simulink model "ErlangSEIRv2_4"  (R2019b)
settings: Solver=VariableStepAuto  StartTime=0.0  StopTime=365  FixedStep=1/24  RelTol=1e-12
undefined symbols (not defined in the file or in its folder): sigbuilder_block
libraries: simulink x2
settings Model: OrderedModelArguments=off  Creator=Alex  LastModifiedBy=Alex

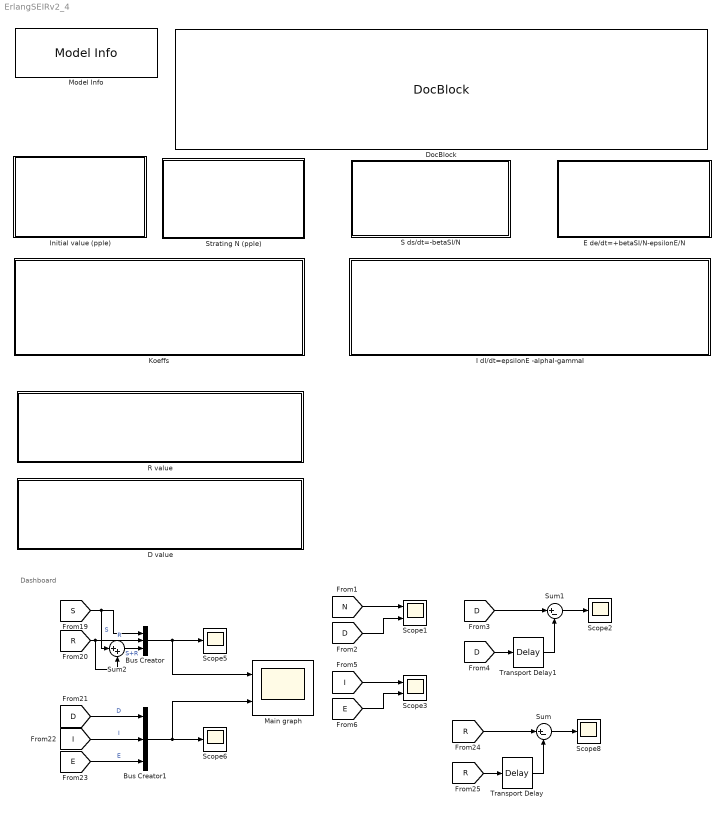
== system ErlangSEIRv2_4 ==
  note: Dashboard
  Bus Creator : BusCreator  Inputs=3
  Bus Creator1 : BusCreator  Inputs=3
  D value : Subsystem
  DocBlock : simulink/Model-Wide Utilities/DocBlock  DocumentType=Text
      content=|
      | Классическая SEIR модель с учетом рождаемости и естественной смертности
      |
      | Учитываются колебания r0 за сутки (часовые ритмы), недельные, месячные (30) дней, и квартальные
      | Ритмы моделируются через синусоиды соответствующего периода (1, 7, 30, 120)
      |
      | Подключен нормально распределенный источник случайностей, частота генерации чисел - 1 день
      |
      | Малое население 1470
      |
      | Учтены ограничительные меры (переключением поправок в Signal Builder)
      | вторая волна не моделируется ввиду исчерпания населения???
      |
      | Для статьи в Резекне 2021
      |
      | На базе этой модели строятся последующие вариации
  E de/dt=+betaSI/N-epsilonE/N : Subsystem
  I dI/dt=epsilonE -alphaI-gammaI : Subsystem
  Initial value (pple) : Subsystem
  Koeffs : Subsystem
  Main graph : Scope  NumInputPorts=2
  Model Info : simulink/Model-Wide Utilities/Model Info  Frame=on  DisplayStringWithTags=|  HorizontalTextAlignment=Left  LeftAlignmentValue=0.02
      | Информация
      | %<Created>
      | %<ModelVersion>
      | %<Description>
  R value : Subsystem
  S ds/dt=-betaSI/N : Subsystem
  Scope1 : Scope  NumInputPorts=2
  Scope{2,5..6,8} (4 alike) : Scope
  Scope3 : Scope  NumInputPorts=2
  Strating N (pple) : Subsystem
  Sum : Sum  Inputs=|+-
  Sum1 : Sum  Inputs=|+-
  Sum2 : Sum  Inputs=|++
  Transport Delay : TransportDelay
  Transport Delay1 : TransportDelay
  wires:
  [S] -> Sum2/1, Bus Creator/1  "S"
  [R] -> Sum2/2, Bus Creator/2  "R"
  [D] -> Bus Creator1/1  "D"
  [I] -> Bus Creator1/2  "I"
  [E] -> Bus Creator1/3  "E"
  Bus Creator/1 -> Main graph/1, Scope5/1
  Bus Creator1/1 -> Main graph/2, Scope6/1
  [R] -> Transport Delay/1
  [R] -> Sum/1
  Transport Delay/1 -> Sum/2
  Sum/1 -> Scope8/1
  [N] -> Scope1/1
  [D] -> Scope1/2
  Sum1/1 -> Scope2/1
  Transport Delay1/1 -> Sum1/2
  [D] -> Sum1/1
  [D] -> Transport Delay1/1
  Sum2/1 -> Bus Creator/3  "S+R"
  [E] -> Scope3/2
  [I] -> Scope3/1

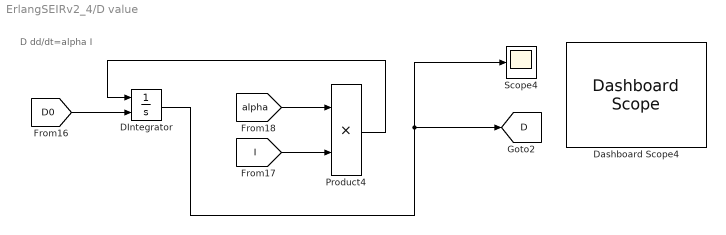
== system ErlangSEIRv2_4/D value ==
  note: D dd/dt=alpha I
  DIntegrator : Integrator  InitialConditionSource=external
  Dashboard Scope4 : DashboardScope  Ymax=150e6
  Product4 : Product  Inputs=**
  Scope4 : Scope
  tag scope: D=global
  wires:
  DIntegrator/1 -> [D], Scope4/1
  [I] -> Product4/2
  [alpha] -> Product4/1
  Product4/1 -> DIntegrator/1
  [D0] -> DIntegrator/2

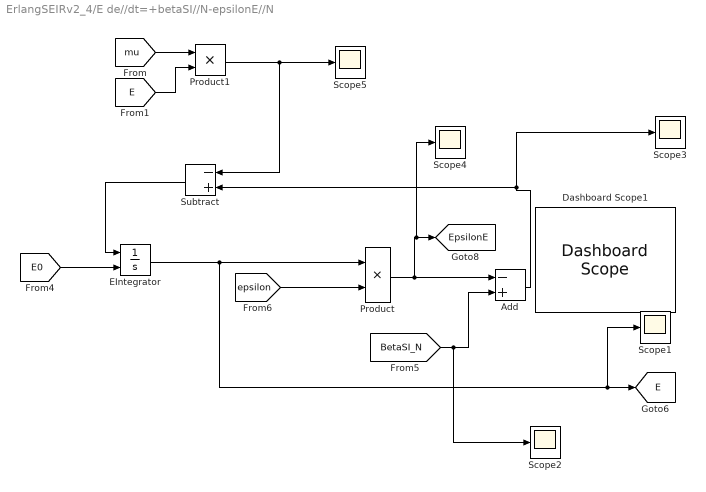
== system ErlangSEIRv2_4/E de//dt=+betaSI//N-epsilonE//N ==
  Add : Sum  Inputs=-+
  Dashboard Scope1 : DashboardScope
  EIntegrator : Integrator  InitialConditionSource=external
  Product : Product  Inputs=**
  Product1 : Product
  Scope{1..5} (5 alike) : Scope
  Subtract : Sum  Inputs=-+
  tag scope: E=global, EpsilonE=global
  wires:
  EIntegrator/1 -> Scope1/1, [E], Product/1
  [BetaSI_N] -> Scope2/1, Add/2
  Add/1 -> Subtract/2, Scope3/1
  [epsilon] -> Product/2
  Product/1 -> Scope4/1, [EpsilonE], Add/1
  [E0] -> EIntegrator/2
  [mu] -> Product1/1
  [E] -> Product1/2
  Subtract/1 -> EIntegrator/1
  Product1/1 -> Scope5/1, Subtract/1

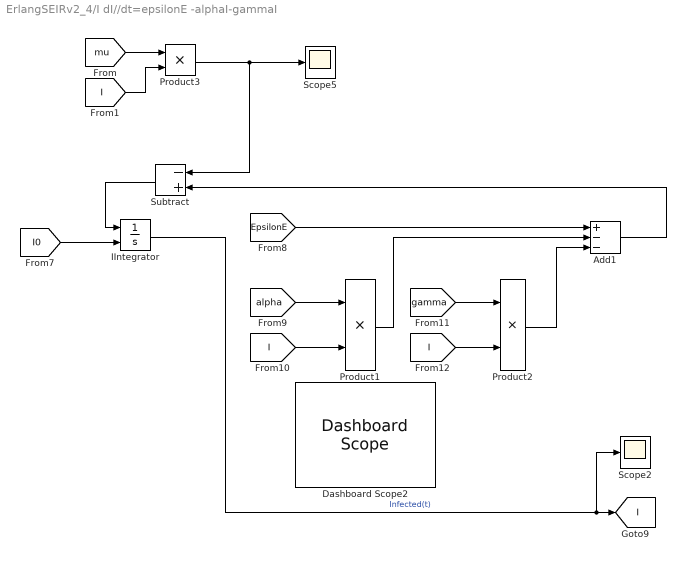
== system ErlangSEIRv2_4/I dI//dt=epsilonE -alphaI-gammaI ==
  Add1 : Sum  Inputs=+--
  Dashboard Scope2 : DashboardScope  Ymax=150e6
  IIntegrator : Integrator  InitialConditionSource=external
  Product1 : Product  Inputs=**
  Product2 : Product  Inputs=**
  Product3 : Product
  Scope2 : Scope
  Scope5 : Scope
  Subtract : Sum  Inputs=-+
  tag scope: I=global
  wires:
  [gamma] -> Product2/1
  Product2/1 -> Add1/3
  [EpsilonE] -> Add1/1
  [alpha] -> Product1/1
  Product1/1 -> Add1/2
  IIntegrator/1 -> [I], Scope2/1  "Infected(t)"
  [I] -> Product1/2
  Add1/1 -> Subtract/2
  [I] -> Product2/2
  [I0] -> IIntegrator/2
  [I] -> Product3/2
  Product3/1 -> Scope5/1, Subtract/1
  [mu] -> Product3/1
  Subtract/1 -> IIntegrator/1

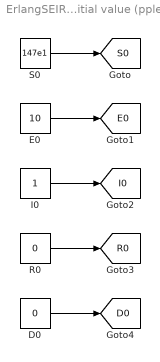
== system ErlangSEIRv2_4/Initial value (pple) ==
  D0 : Constant  Value=0
  E0 : Constant  Value=10
  I0 : Constant
  R0 : Constant  Value=0
  S0 : Constant  Value=147e1
  tag scope: D0=global, E0=global, I0=global, R0=global, S0=global
  wires:
  S0/1 -> [S0]
  I0/1 -> [I0]
  D0/1 -> [D0]
  E0/1 -> [E0]
  R0/1 -> [R0]

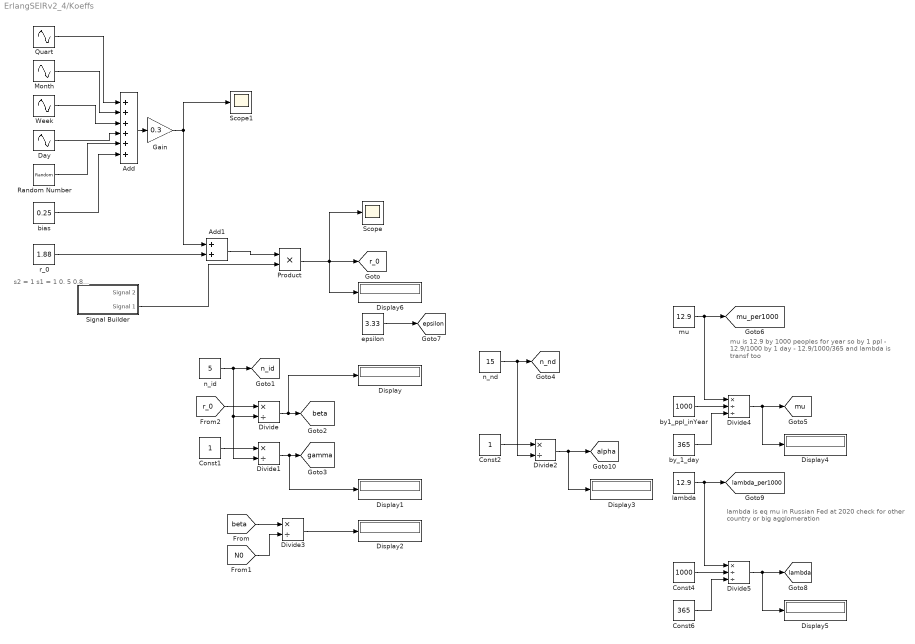
== system ErlangSEIRv2_4/Koeffs ==
  note: s2 = 1
      | s1 = 1 0. 5 0.8...
  note: lambda is eq mu in Russian Fed at 2020
      | check for other country or big agglomeration
  note: mu is 12.9 by 1000 peoples for year
      | so by 1 ppl - 12.9/1000
      | by 1 day - 12.9/1000/365
      | and lambda is transf too
  Add : Sum  Inputs=++++++
  Add1 : Sum
  Const1 : Constant
  Const2 : Constant
  Const4 : Constant  Value=1000
  Const6 : Constant  Value=365
  Day : Sin  Amplitude=0.12  Frequency=2*pi/7  SampleTime=0
  Display{,1..6} (7 alike) : Display
  Divide{,1..3} (4 alike) : Product  Inputs=*/
  Divide4 : Product  Inputs=*//
  Divide5 : Product  Inputs=*//
  Gain : Gain  Gain=0.3
  Month : Sin  Amplitude=0.12  Frequency=2*pi/30  SampleTime=0
  Product : Product
  Quart : Sin  Amplitude=0.12  Frequency=2*pi/120  SampleTime=0
  Random Number : RandomNumber  Variance=0.0144  SampleTime=1
  Scope : Scope
  Scope1 : Scope
  Signal Builder : Subsystem  Tag=STV Subsys  LoadFcn=sigbuilder_block('load');  StartFcn=sigbuilder_block('start');  StopFcn=sigbuilder_block('stop');  ClipboardFcn=sigbuilder_block('clipboard');  mask(Sigbuilder block){tuvar=[0:10]}
      mask help: Simulink:masks:SigbuilderBlock_MD
      mask init:
      | if ~strcmp(get_param(bdroot(gcbh),'SimulationStatus'),'stopped') tuvar = sigbuilder_block('maskInit'); end
      settings: CopyFcn=sigbuilder_block('copy');  DeleteFcn=sigbuilder_block('delete');  ModelCloseFcn=sigbuilder_block('modelClose');  PreSaveFcn=sigbuilder_block('preSave');  PauseFcn=sigbuilder_block('pause');  ContinueFcn=sigbuilder_block('continue');  NameChangeFcn=sigbuilder_block('namechange');  OpenFcn=sigbuilder_block('open',[437.6 199.2 550.4 400 ]);  CloseFcn=sigbuilder_block('close');
      mask Display: plot(0, 0, 100, 100,[2, 2, 32, 32, 2], [68, 8, 8, 68, 68],[32, 2], [38, 38], [32, 19, 2],[53, 60, 44], [32, 17, 17, 2],[16, 16, 31, 31]);txt = getActiveGroup(gcbh);text(2, 100, txt,'verticalAlignment', 'top');
  Week : Sin  Amplitude=0.12  Frequency=2*pi/7  SampleTime=0
  bias : Constant  Value=0.25
  by1_ppl_inYear : Constant  Value=1000
  by_1_day : Constant  Value=365
  epsilon : Constant  Value=3.33
  lambda : Constant  Value=12.9
  mu : Constant  Value=12.9
  n_id : Constant  Value=5
  n_nd : Constant  Value=15
  r_0 : Constant  Value=1.88
  tag scope: alpha=global, beta=global, epsilon=global, gamma=global, lambda=global, lambda_per1000=global, mu=global, mu_per1000=global, n_id=global, n_nd=global, r_0=global
  wires:
  Divide1/1 -> Display1/1, [gamma]
  n_id/1 -> Divide1/2, Divide/2, [n_id]
  Divide/1 -> Display/1, [beta]
  Const1/1 -> Divide1/1
  epsilon/1 -> [epsilon]
  Const2/1 -> Divide2/1
  Divide2/1 -> Display3/1, [alpha]
  n_nd/1 -> [n_nd], Divide2/2
  [beta] -> Divide3/1
  [N0] -> Divide3/2
  Divide3/1 -> Display2/1
  mu/1 -> Divide4/1, [mu_per1000]
  Divide4/1 -> [mu], Display4/1
  by1_ppl_inYear/1 -> Divide4/2
  Const4/1 -> Divide5/2
  Divide5/1 -> Display5/1, [lambda]
  lambda/1 -> [lambda_per1000], Divide5/1
  Const6/1 -> Divide5/3
  by_1_day/1 -> Divide4/3
  r_0/1 -> Add1/2
  Product/1 -> Scope/1, Display6/1, [r_0]
  [r_0] -> Divide/1
  Quart/1 -> Add/1
  Month/1 -> Add/2
  Week/1 -> Add/3
  Day/1 -> Add/4
  Add/1 -> Gain/1
  Add1/1 -> Product/1
  Random Number/1 -> Add/5
  bias/1 -> Add/6
  Gain/1 -> Scope1/1, Add1/1
  Signal Builder/2(Signal 1) -> Product/2

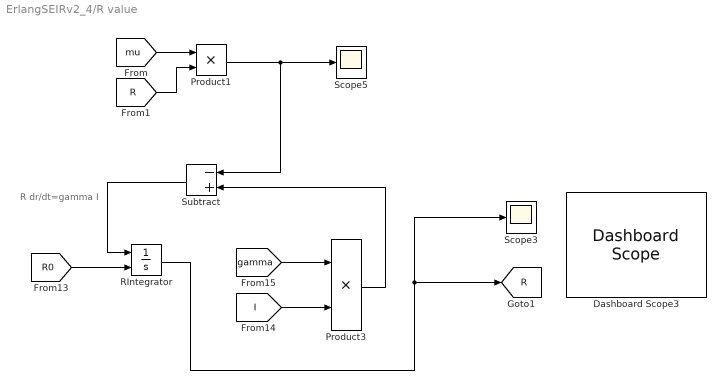
== system ErlangSEIRv2_4/R value ==
  note: R dr/dt=gamma I
  Dashboard Scope3 : DashboardScope
  Product1 : Product
  Product3 : Product  Inputs=**
  RIntegrator : Integrator  InitialConditionSource=external
  Scope3 : Scope
  Scope5 : Scope
  Subtract : Sum  Inputs=-+
  tag scope: R=global
  wires:
  Product3/1 -> Subtract/2
  [I] -> Product3/2
  [R0] -> RIntegrator/2
  [gamma] -> Product3/1
  RIntegrator/1 -> Scope3/1, [R]
  [R] -> Product1/2
  Product1/1 -> Scope5/1, Subtract/1
  [mu] -> Product1/1
  Subtract/1 -> RIntegrator/1

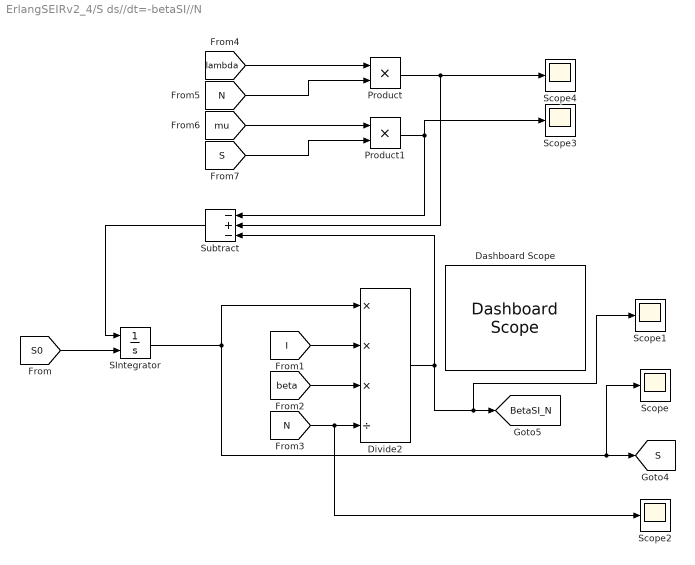
== system ErlangSEIRv2_4/S ds//dt=-betaSI//N ==
  Dashboard Scope : DashboardScope  Ymax=150e6
  Divide2 : Product  Inputs=***/
  Product : Product
  Product1 : Product
  SIntegrator : Integrator  InitialConditionSource=external
  Scope{,1..4} (5 alike) : Scope
  Subtract : Sum  Inputs=-+-
  tag scope: BetaSI_N=global, S=global
  wires:
  Divide2/1 -> Subtract/3, Scope1/1, [BetaSI_N]
  SIntegrator/1 -> Scope/1, [S], Divide2/1
  [N] -> Scope2/1, Divide2/4
  [beta] -> Divide2/3
  [I] -> Divide2/2
  [S0] -> SIntegrator/2
  Subtract/1 -> SIntegrator/1
  [mu] -> Product1/1
  [S] -> Product1/2
  Product1/1 -> Subtract/1, Scope3/1
  [lambda] -> Product/1
  [N] -> Product/2
  Product/1 -> Scope4/1, Subtract/2

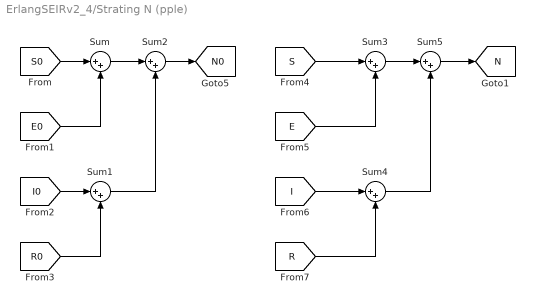
== system ErlangSEIRv2_4/Strating N (pple) ==
  Sum{,1..5} (6 alike) : Sum  Inputs=|++
  tag scope: N0=global, N=global
  wires:
  [I0] -> Sum1/1
  [S0] -> Sum/1
  [E0] -> Sum/2
  [R0] -> Sum1/2
  Sum2/1 -> [N0]
  Sum1/1 -> Sum2/2
  Sum/1 -> Sum2/1
  [S] -> Sum3/1
  [E] -> Sum3/2
  [I] -> Sum4/1
  [R] -> Sum4/2
  Sum3/1 -> Sum5/1
  Sum4/1 -> Sum5/2
  Sum5/1 -> [N]

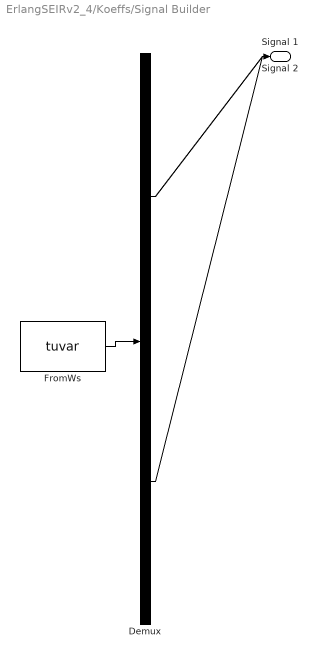
== system ErlangSEIRv2_4/Koeffs/Signal Builder ==
  Demux : Demux  Tag=STV Demux  Outputs=2
  FromWs : FromWorkspace  Tag=STV FromWs  VariableName=tuvar  SampleTime=0
      SigBuilderData=|
      | common.afterFinalStr = 'Extrapolate'
      | common.sampleTime = 0
      | dataSet.timeRange = [0 365]
      | dataSet.name = 'Group 1'
      | sbobj.Groups.Name = 'Group 1'
      | sbobj.Groups.Signals(1).Name = 'Signal 2'
      | sbobj.Groups.Signals(1).XData = [0 365]
      | sbobj.Groups.Signals(1).YData = [1 1]
      | sbobj.Groups.Signals(2).Name = 'Signal 1'
      | sbobj.Groups.Signals(2).XData = [0 80 85 125 126 186 187 365]
      | sbobj.Groups.Signals(2).YData = [1 1 0.5 0.5 0.8 0.8 0.85 0.85]
      | sbobj.Groups.TimeRange = [0 365]
  Signal 2 : Outport  Tag=STV Outport
  Signal 1 : Outport  Tag=STV Outport  Port=2
  wires:
  FromWs/1 -> Demux/1
  Demux/1 -> Signal 2/1
  Demux/2 -> Signal 1/1
